simulink model "adaptive_control_omeraysal2"  (R2023b)
settings: Solver=VariableStepAuto  StartTime=0.0  StopTime=100  FixedStep=0.001  MaxStep=0.001  RelTol=1e-4
settings Model: Creator=sukrunver  LastModifiedBy=melis
settings SolverCC: AlgebraicLoopSolver=TrustRegion
settings SFSimCC: CustomCodeUndefinedFunction=UseInterfaceOnly

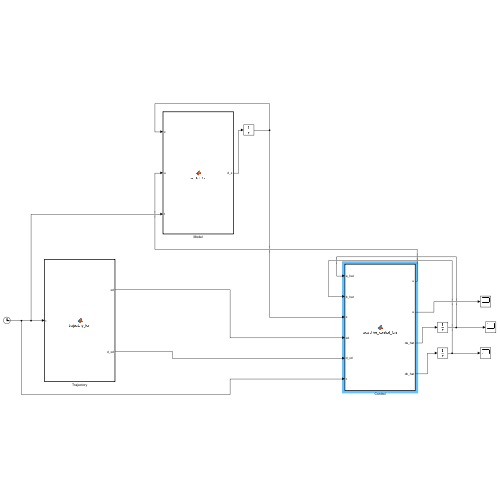
[thumbnail: Simulink's stored preview of the top-level diagram]
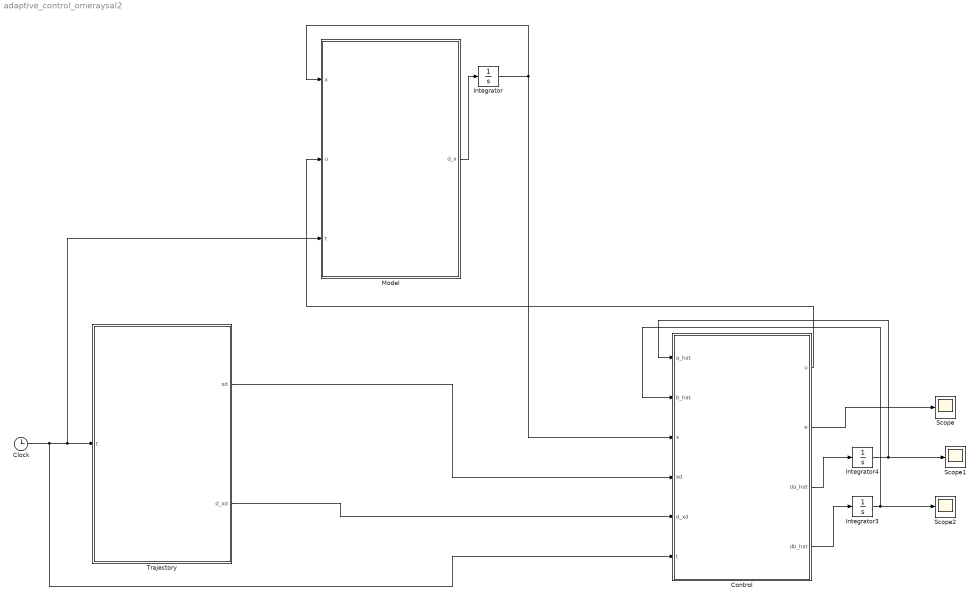
== system adaptive_control_omeraysal2 ==
  Clock : Clock
  Control : MATLAB Function  TreatAsAtomicUnit=on
  Integrator : Integrator
  Integrator3 : Integrator
  Integrator4 : Integrator
  Model : MATLAB Function  TreatAsAtomicUnit=on
  Scope : Scope
  Scope1 : Scope
  Scope2 : Scope
  Trajectory : MATLAB Function  TreatAsAtomicUnit=on
  wires:
  Model/1(d_x) -> Integrator/1
  Control/2(e) -> Scope/1
  Clock/1 -> Control/6(t), Model/3(t), Trajectory/1(t)
  Control/1(u) -> Model/2(u)
  Trajectory/1(xd) -> Control/4(xd)
  Trajectory/2(d_xd) -> Control/5(d_xd)
  Control/3(da_hat) -> Integrator4/1
  Integrator4/1 -> Scope1/1, Control/1(a_hat)
  Control/4(db_hat) -> Integrator3/1
  Integrator3/1 -> Scope2/1, Control/2(b_hat)
  Integrator/1 -> Model/1(x), Control/3(x)

== matlab function adaptive_control_omeraysal2/Trajectory ==
  data: t input; xd output; d_xd output
function [xd, d_xd] = trajectory_fcn(t)
    xd   =  sin(t);
    d_xd =  cos(t);
end

== matlab function adaptive_control_omeraysal2/Model ==
  data: x input; d_x output; u input; t input
function d_x = model_fcn(x, u, t)
    a_true = 2.0;
    b_true = 1.5;
    f_xt   = a_true * x^2 + b_true * cos(t);
    d_x    = f_xt + u;
end

== matlab function adaptive_control_omeraysal2/Control ==
  settings: updateMethod=DISCRETE
  data: a_hat input; b_hat input; u output; x input; xd input; d_xd input; e output; t input; da_hat output; db_hat output
function [u, e, da_hat, db_hat] = adaptive_control_fcn( a_hat, b_hat, x, xd, d_xd, t)

    k = 5;

    gamma_a = 1;
    gamma_b = 1;

    e = xd - x;

    phi_1 = x^2;
    phi_2 = cos(t);

    f_hat = a_hat*phi_1 + b_hat*phi_2;

    u = d_xd - f_hat + k*e;

    da_hat = -gamma_a * phi_1 * e;
    db_hat = -gamma_b * phi_2 * e;

end
